simulink model "Lateral Dynamics Improvement using Active Rear Wing Control"  (R2018b)
settings: Solver=FixedStepAuto  StartTime=0.0  StopTime=10.0  FixedStep=0.005  RelTol=1e-3
settings Model: Creator=12779  LastModifiedBy=12779

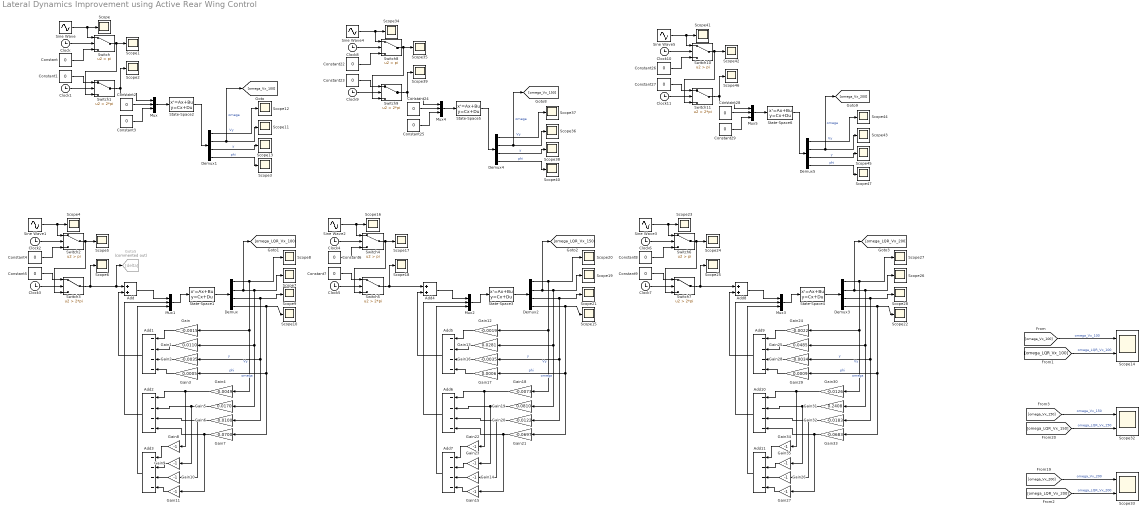
== system Lateral Dynamics Improvement using Active Rear Wing Control ==
  Add : Sum
  Add{1..3,5..7,9..11} (9 alike) : Sum  Inputs=----
  Add4 : Sum
  Add8 : Sum
  Clock{,1..11} (12 alike) : Clock
  Constant{,1..9,22..29} (18 alike) : Constant  Value=0
  Demux{,1..5} (6 alike) : Demux
  Gain : Gain  Gain=-0.0015
  Gain1 : Gain  Gain=0.0110
  Gain{8..11,14..15,22..23,26..27,34..35} (12 alike) : Gain  Gain=-1
  Gain12 : Gain  Gain=-0.0019
  Gain13 : Gain  Gain=0.0281
  Gain16 : Gain  Gain=-0.0035
  Gain17 : Gain  Gain=0.0006
  Gain18 : Gain  Gain=-0.0073
  Gain19 : Gain  Gain=0.0810
  Gain2 : Gain  Gain=-0.0035
  Gain20 : Gain  Gain=-0.0122
  Gain21 : Gain  Gain=-0.0697
  Gain24 : Gain  Gain=-0.0022
  Gain25 : Gain  Gain=0.0485
  Gain28 : Gain  Gain=-0.0034
  Gain29 : Gain  Gain=0.0009
  Gain3 : Gain  Gain=0.0005
  Gain30 : Gain  Gain=-0.0126
  Gain31 : Gain  Gain=0.2408
  Gain32 : Gain  Gain=-0.0183
  Gain33 : Gain  Gain=-0.0683
  Gain4 : Gain  Gain=-0.0049
  Gain5 : Gain  Gain=0.0170
  Gain6 : Gain  Gain=-0.0100
  Gain7 : Gain  Gain=-0.0700
  Goto5 : Goto  Commented=on  GotoTag=delta
  Mux{,1..5} (6 alike) : Mux  Inputs=3
  Scope{,1..13,15..28,34..47} (42 alike) : Scope
  Scope14 : Scope  NumInputPorts=2
  Scope32 : Scope  NumInputPorts=2
  Scope33 : Scope  NumInputPorts=2
  Sine Wave{,1..5} (6 alike) : Sin  Amplitude=0.03  Frequency=2  SampleTime=0
  State-Space1 : StateSpace  A=[-1.7192 -27.6106 0 0;0.1440 -3.7551 0 0;1 0 0 0;0 1 0 0]  B=[23.9013 0 0;30.4741 0.0454 -0.0454;0 0 0;0 0 0]  C=[1 0 0 0;0 1 0 0;0 0 1 0;0 0 0 1]  D=[0 0 0;0 0 0;0 0 0;0 0 0]  InitialCondition=0
  State-Space2 : StateSpace  A=[-1.7192 -27.6106 0 0;0.1440 -3.7551 0 0;1 0 0 0;0 1 0 0]  B=[23.9013 0 0;30.4741 0.0454 -0.0454;0 0 0;0 0 0]  C=[1 0 0 0;0 1 0 0;0 0 1 0;0 0 0 1]  D=[0 0 0;0 0 0;0 0 0;0 0 0]  InitialCondition=0
  State-Space3 : StateSpace  A=[-1.1464 -41.5470 0 0;0.0960 -2.5040 0 0;1 0 0 0;0 1 0 0]  B=[23.9013 0 0;30.4741 0.1021 -0.1021;0 0 0;0 0 0]  C=[1 0 0 0;0 1 0 0;0 0 1 0;0 0 0 1]  D=[0 0 0;0 0 0;0 0 0;0 0 0]  InitialCondition=0
  State-Space4 : StateSpace  A=[-0.8596 -55.4753 0 0;0.0720 -1.8776 0 0;1 0 0 0;0 1 0 0]  B=[23.9013 0 0;30.4741 0.1815 -0.1815;0 0 0;0 0 0]  C=[1 0 0 0;0 1 0 0;0 0 1 0;0 0 0 1]  D=[0 0 0;0 0 0;0 0 0;0 0 0]  InitialCondition=0
  State-Space5 : StateSpace  A=[-1.1464 -41.5470 0 0;0.0960 -2.5040 0 0;1 0 0 0;0 1 0 0]  B=[23.9013 0 0;30.4741 0.1021 -0.1021;0 0 0;0 0 0]  C=[1 0 0 0;0 1 0 0;0 0 1 0;0 0 0 1]  D=[0 0 0;0 0 0;0 0 0;0 0 0]  InitialCondition=0
  State-Space6 : StateSpace  A=[-0.8596 -55.4753 0 0;0.0720 -1.8776 0 0;1 0 0 0;0 1 0 0]  B=[23.9013 0 0;30.4741 0.1815 -0.1815;0 0 0;0 0 0]  C=[1 0 0 0;0 1 0 0;0 0 1 0;0 0 0 1]  D=[0 0 0;0 0 0;0 0 0;0 0 0]  InitialCondition=0
  Switch{,2,4,6,8,10} (6 alike) : Switch  Criteria=u2 > Threshold  Threshold=pi
  Switch{1,3,5,7,9,11} (6 alike) : Switch  Criteria=u2 > Threshold  Threshold=2*pi
  wires:
  Sine Wave/1 -> Scope/1, Switch/1
  Clock/1 -> Switch/2
  Switch/1 -> Switch1/3, Scope1/1
  Constant/1 -> Switch/3
  Clock1/1 -> Switch1/2
  Constant1/1 -> Switch1/1
  Switch1/1 -> Mux/1, Scope2/1
  Constant2/1 -> Mux/2
  Constant3/1 -> Mux/3
  Constant5/1 -> Switch3/1
  Switch3/1 -> Goto5/1, Add/1, Scope6/1
  Mux1/1 -> State-Space1/1
  Clock3/1 -> Switch3/2
  Constant4/1 -> Switch2/3
  Sine Wave1/1 -> Scope4/1, Switch2/1
  Clock2/1 -> Switch2/2
  Switch2/1 -> Switch3/3, Scope5/1
  State-Space1/1 -> Demux/1
  Add/1 -> Mux1/1
  Gain/1 -> Add1/1
  Gain1/1 -> Add1/2
  Gain2/1 -> Add1/3
  Gain3/1 -> Add1/4
  Add1/1 -> Add/2
  Add2/1 -> Mux1/2
  Gain7/1 -> Gain11/1, Add2/4
  Gain6/1 -> Gain10/1, Add2/3
  Gain5/1 -> Gain9/1, Add2/2
  Gain4/1 -> Gain8/1, Add2/1
  Demux/2 -> Scope7/1, Gain5/1, Gain1/1, [omega_LQR_Vx_100]  "omega"
  Demux/1 -> Scope8/1, Gain4/1, Gain/1  "Vy"
  Demux/3 -> Gain6/1, Gain2/1, Scope9/1  "y"
  Demux/4 -> Gain7/1, Gain3/1, Scope10/1  "phi"
  Gain8/1 -> Add3/1
  Add3/1 -> Mux1/3
  Demux1/4 -> Scope3/1  "phi"
  Demux1/3 -> Scope13/1  "y"
  Demux1/1 -> Scope12/1  "Vy"
  Demux1/2 -> [omega_Vx_100], Scope11/1  "omega"
  State-Space2/1 -> Demux1/1
  Mux/1 -> State-Space2/1
  Gain9/1 -> Add3/2
  Gain10/1 -> Add3/3
  Gain11/1 -> Add3/4
  Constant6/1 -> Switch4/3
  Sine Wave2/1 -> Scope16/1, Switch4/1
  Mux2/1 -> State-Space3/1
  Clock5/1 -> Switch5/2
  Constant7/1 -> Switch5/1
  Demux2/3 -> Gain20/1, Gain16/1, Scope21/1  "y"
  Gain22/1 -> Add7/1
  Gain18/1 -> Gain22/1, Add6/1
  Gain19/1 -> Gain23/1, Add6/2
  Gain21/1 -> Gain15/1, Add6/4
  Gain20/1 -> Gain14/1, Add6/3
  Clock4/1 -> Switch4/2
  Gain12/1 -> Add5/1
  Demux2/2 -> Scope19/1, Gain19/1, Gain13/1, [omega_LQR_Vx_150]  "omega"
  Gain17/1 -> Add5/4
  Gain13/1 -> Add5/2
  Demux2/1 -> Scope20/1, Gain18/1, Gain12/1  "Vy"
  Gain16/1 -> Add5/3
  Gain14/1 -> Add7/3
  Add5/1 -> Add4/2
  Gain15/1 -> Add7/4
  Gain23/1 -> Add7/2
  Demux2/4 -> Gain21/1, Gain17/1, Scope15/1  "phi"
  Add6/1 -> Mux2/2
  Switch5/1 -> Add4/1, Scope18/1
  Switch4/1 -> Switch5/3, Scope17/1
  Add4/1 -> Mux2/1
  Add7/1 -> Mux2/3
  State-Space3/1 -> Demux2/1
  State-Space4/1 -> Demux3/1
  Add11/1 -> Mux3/3
  Add8/1 -> Mux3/1
  Switch6/1 -> Scope24/1, Switch7/3
  Switch7/1 -> Scope25/1, Add8/1
  Add10/1 -> Mux3/2
  Demux3/4 -> Scope22/1, Gain29/1, Gain33/1  "phi"
  Gain35/1 -> Add11/2
  Gain27/1 -> Add11/4
  Add9/1 -> Add8/2
  Gain26/1 -> Add11/3
  Gain28/1 -> Add9/3
  Demux3/1 -> Gain24/1, Gain30/1, Scope27/1  "Vy"
  Gain25/1 -> Add9/2
  Gain29/1 -> Add9/4
  Demux3/2 -> [omega_LQR_Vx_200], Gain25/1, Gain31/1, Scope26/1  "omega"
  Gain24/1 -> Add9/1
  Clock6/1 -> Switch6/2
  Gain32/1 -> Add10/3, Gain26/1
  Gain33/1 -> Add10/4, Gain27/1
  Gain31/1 -> Add10/2, Gain35/1
  Gain30/1 -> Add10/1, Gain34/1
  Gain34/1 -> Add11/1
  Demux3/3 -> Scope28/1, Gain28/1, Gain32/1  "y"
  Constant9/1 -> Switch7/1
  Clock7/1 -> Switch7/2
  Mux3/1 -> State-Space4/1
  Sine Wave3/1 -> Switch6/1, Scope23/1
  Constant8/1 -> Switch6/3
  Mux4/1 -> State-Space5/1
  State-Space5/1 -> Demux4/1
  Demux4/2 -> Scope36/1, [omega_Vx_150]  "omega"
  Demux4/1 -> Scope37/1  "Vy"
  Demux4/3 -> Scope38/1  "y"
  Demux4/4 -> Scope40/1  "phi"
  Constant25/1 -> Mux4/3
  Constant24/1 -> Mux4/2
  Switch9/1 -> Scope39/1, Mux4/1
  Constant23/1 -> Switch9/1
  Clock9/1 -> Switch9/2
  Constant22/1 -> Switch8/3
  Switch8/1 -> Scope35/1, Switch9/3
  Clock8/1 -> Switch8/2
  Sine Wave4/1 -> Switch8/1, Scope34/1
  Sine Wave5/1 -> Scope41/1, Switch10/1
  Clock10/1 -> Switch10/2
  Switch10/1 -> Switch11/3, Scope42/1
  Constant26/1 -> Switch10/3
  Clock11/1 -> Switch11/2
  Constant27/1 -> Switch11/1
  Switch11/1 -> Mux5/1, Scope46/1
  Constant28/1 -> Mux5/2
  Constant29/1 -> Mux5/3
  Demux5/4 -> Scope47/1  "phi"
  Demux5/3 -> Scope45/1  "y"
  Demux5/1 -> Scope44/1  "Vy"
  Demux5/2 -> [omega_Vx_200], Scope43/1  "omega"
  State-Space6/1 -> Demux5/1
  Mux5/1 -> State-Space6/1
  [omega_Vx_150] -> Scope32/1  "omega_Vx_150"
  [omega_LQR_Vx_200] -> Scope33/2  "omega_LQR_Vx_200"
  [omega_LQR_Vx_150] -> Scope32/2  "omega_LQR_Vx_150"
  [omega_Vx_200] -> Scope33/1  "omega_Vx_200"
  [omega_Vx_100] -> Scope14/1  "omega_Vx_100"
  [omega_LQR_Vx_100] -> Scope14/2  "omega_LQR_Vx_100"
